simulink model "sim_tank_2_PI"  (R2016b)
settings: Solver=VariableStepAuto  StartTime=0.0  StopTime=10.0  RelTol=1e-3
values from neighbouring files (symbols this model uses):
  Ao1 = pi * Do1^2 / 4    (= 0.17813934812)    [setup_tanks_parameters.m]
  Ao2 = pi * Do2^2 / 4    (= 0.17813934812)    [setup_tanks_parameters.m]
  At1 = pi * Dt1^2 / 4    (= 15.5179165474)    [setup_tanks_parameters.m]
  At2 = pi * Dt2^2 / 4    (= 15.5179165474)    [setup_tanks_parameters.m]
  g = 981    [setup_tanks_parameters.m]
  Ki_1 = Ki1_pp    [d_tanks_1.m]    (also in setup_lab_tanks.m = 0)
  Ki_2 = Ki2_pp    [d_tanks_2.m]    (also in d_tanks_3.m = K(3); setup_lab_tanks.m = 0)
  Kp = 3.3    [setup_tanks_parameters.m]
  Kp_1 = Kp1_pp    [d_tanks_1.m]    (also in d_tanks_3.m = K(1); setup_lab_tanks.m = 0)
  Kp_2 = Kp2_pp    [d_tanks_2.m]    (also in d_tanks_3.m = K(2); setup_lab_tanks.m = 0)
  L20 = L0    [d_tanks_2.m]    (also in setup_lab_tanks.m = 10)
  LR_1_MAX = 25    [setup_lab_tanks.m]
  MAX_L1_WDUP = 3    [setup_lab_tanks.m]
  MAX_L2_WDUP = 3    [setup_lab_tanks.m]
  TS = 35    [setup_lab_tanks.m]
  VMAX_AMP = 22    [setup_tanks_parameters.m]
settings Model: Creator=yuthon  LastModifiedBy=yuthon

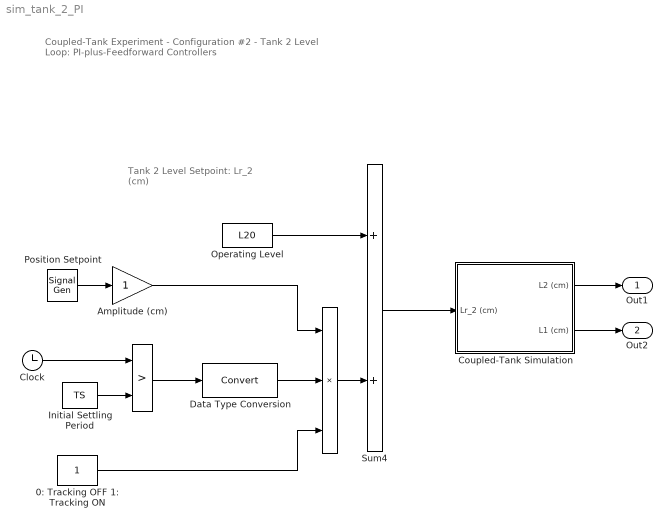
== system sim_tank_2_PI ==
  note: Coupled-Tank Experiment
      | - Configuration #2 -
      | Tank 2 Level Loop:
      | PI-plus-Feedforward Controllers
  note: Tank 2 Level Setpoint:
      | Lr_2 (cm)
  "   " : Product  Inputs=3  SaturateOnIntegerOverflow=on  RndMeth=Zero  InputSameDT=on  OutDataTypeStr=Inherit: Same as first input
  "    " : RelationalOperator  Operator=>  RndMeth=Nearest  InputSameDT=on
  0: Tracking OFF 1: Tracking ON : Constant
  Amplitude (cm) : Gain  SaturateOnIntegerOverflow=on  OutDataTypeStr=Inherit: Same as input  ParamDataTypeStr=Inherit: Same as input
  Clock : Clock
  Coupled-Tank Simulation : Subsystem
  Data Type Conversion : DataTypeConversion
  Initial Settling Period : Constant  Value=TS
  Operating Level : Constant  Value=L20
  Position Setpoint : SignalGenerator  WaveForm=square  Frequency=0.018
  Sum4 : Sum  SaturateOnIntegerOverflow=on  InputSameDT=on  OutDataTypeStr=Inherit: Same as first input
  Out1 : Outport  SignalName=L2  InitialOutput=0
  Out2 : Outport  Port=2  SignalName=L1  InitialOutput=0
  wires:
  Position Setpoint/1 -> Amplitude (cm)/1
  0: Tracking OFF 1: Tracking ON/1 -> "   "/3
  "   "/1 -> Sum4/2
  Operating Level/1 -> Sum4/1
  Initial Settling Period/1 -> "    "/2
  Clock/1 -> "    "/1
  Amplitude (cm)/1 -> "   "/1
  Coupled-Tank Simulation/2(L1 (cm)) -> Out2/1
  "    "/1 -> Data Type Conversion/1
  Data Type Conversion/1 -> "   "/2
  Sum4/1 -> Coupled-Tank Simulation/1(Lr_2 (cm))
  Coupled-Tank Simulation/1(L2 (cm)) -> Out1/1

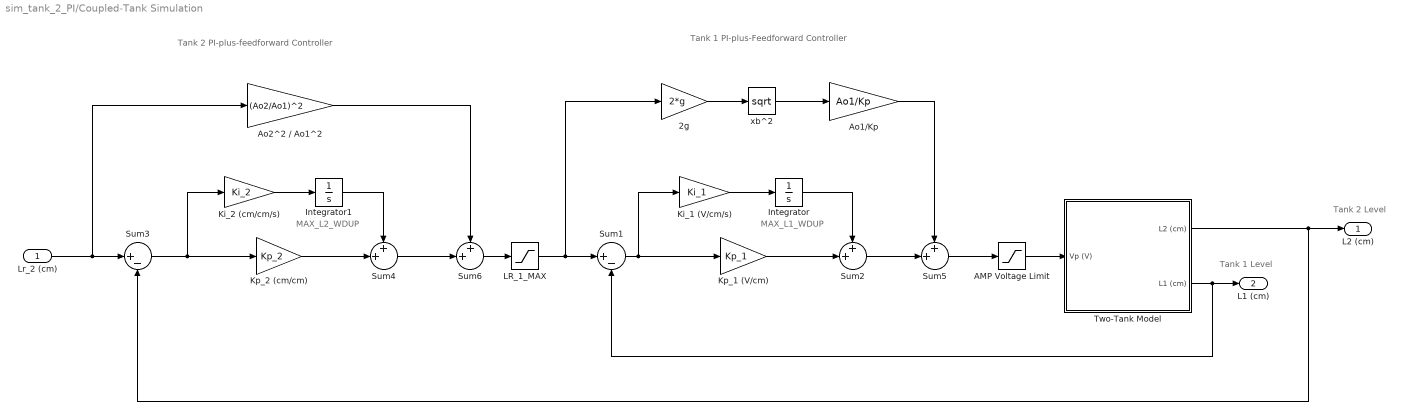
== system sim_tank_2_PI/Coupled-Tank Simulation ==
  note: Tank 1
      | PI-plus-Feedforward Controller
  note: Tank 2
      | PI-plus-feedforward Controller
  note: MAX_L2_WDUP
  note: Tank 1 Level
  note: Tank 2 Level
  note: MAX_L1_WDUP
  Lr_2 (cm) : Inport
  2g : Gain  Gain=2*g  SaturateOnIntegerOverflow=on  OutDataTypeStr=Inherit: Same as input  ParamDataTypeStr=Inherit: Same as input
  AMP Voltage Limit : Saturate  UpperLimit=VMAX_AMP  LowerLimit=0
  Ao1/Kp : Gain  Gain=Ao1/Kp  SaturateOnIntegerOverflow=on  OutDataTypeStr=Inherit: Same as input  ParamDataTypeStr=Inherit: Same as input
  Ao2^2 / Ao1^2 : Gain  Gain=(Ao2/Ao1)^2  SaturateOnIntegerOverflow=on  OutDataTypeStr=Inherit: Same as input  ParamDataTypeStr=Inherit: Same as input
  Integrator : Integrator  LimitOutput=on  UpperSaturationLimit=MAX_L1_WDUP  LowerSaturationLimit=- MAX_L1_WDUP
  Integrator1 : Integrator  LimitOutput=on  UpperSaturationLimit=MAX_L2_WDUP  LowerSaturationLimit=- MAX_L2_WDUP
  Ki_1 (V/cm/s) : Gain  Gain=Ki_1  SaturateOnIntegerOverflow=on  OutDataTypeStr=Inherit: Same as input  ParamDataTypeStr=Inherit: Same as input
  Ki_2 (cm/cm/s) : Gain  Gain=Ki_2  SaturateOnIntegerOverflow=on  OutDataTypeStr=Inherit: Same as input  ParamDataTypeStr=Inherit: Same as input
  Kp_1 (V/cm) : Gain  Gain=Kp_1  SaturateOnIntegerOverflow=on  OutDataTypeStr=Inherit: Same as input  ParamDataTypeStr=Inherit: Same as input
  Kp_2 (cm/cm) : Gain  Gain=Kp_2  SaturateOnIntegerOverflow=on  OutDataTypeStr=Inherit: Same as input  ParamDataTypeStr=Inherit: Same as input
  LR_1_MAX : Saturate  UpperLimit=LR_1_MAX  LowerLimit=0
  Sum1 : Sum  Inputs=|+-  SaturateOnIntegerOverflow=on  InputSameDT=on  OutDataTypeStr=Inherit: Same as first input
  Sum{2,4..6} (4 alike) : Sum  Inputs=++|  SaturateOnIntegerOverflow=on  InputSameDT=on  OutDataTypeStr=Inherit: Same as first input
  Sum3 : Sum  Inputs=|+-  SaturateOnIntegerOverflow=on  InputSameDT=on  OutDataTypeStr=Inherit: Same as first input
  Two-Tank Model : Subsystem
  xb^2 : Math  Operator=sqrt  SaturateOnIntegerOverflow=on
  L2 (cm) : Outport  InitialOutput=0
  L1 (cm) : Outport  Port=2  InitialOutput=0
  wires:
  LR_1_MAX/1 -> 2g/1, Sum1/1
  Lr_2 (cm)/1 -> Ao2^2 / Ao1^2/1, Sum3/1
  Ao2^2 / Ao1^2/1 -> Sum6/1
  Sum6/1 -> LR_1_MAX/1
  Sum4/1 -> Sum6/2
  Integrator1/1 -> Sum4/1
  Kp_2 (cm/cm)/1 -> Sum4/2
  Ki_2 (cm/cm/s)/1 -> Integrator1/1
  Sum3/1 -> Kp_2 (cm/cm)/1, Ki_2 (cm/cm/s)/1
  Two-Tank Model/1(L2 (cm)) -> Sum3/2, L2 (cm)/1
  Two-Tank Model/2(L1 (cm)) -> L1 (cm)/1, Sum1/2
  Ao1/Kp/1 -> Sum5/1
  xb^2/1 -> Ao1/Kp/1
  2g/1 -> xb^2/1
  Sum5/1 -> AMP Voltage Limit/1
  Sum2/1 -> Sum5/2
  AMP Voltage Limit/1 -> Two-Tank Model/1(Vp (V))
  Integrator/1 -> Sum2/1
  Kp_1 (V/cm)/1 -> Sum2/2
  Ki_1 (V/cm/s)/1 -> Integrator/1
  Sum1/1 -> Kp_1 (V/cm)/1, Ki_1 (V/cm/s)/1

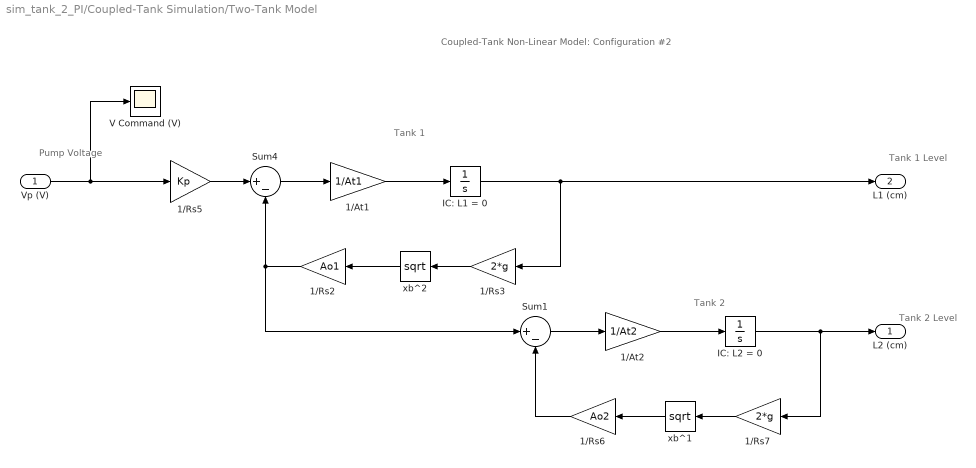
== system sim_tank_2_PI/Coupled-Tank Simulation/Two-Tank Model ==
  note: Pump
      | Voltage
  note: Tank 1 Level
  note: Tank 2 Level
  note: Tank 2
  note: Tank 1
  note: Coupled-Tank Non-Linear Model:
      | Configuration #2
  Vp (V) : Inport
  1/At1 : Gain  Gain=1/At1  SaturateOnIntegerOverflow=on  OutDataTypeStr=Inherit: Same as input  ParamDataTypeStr=Inherit: Same as input
  1/At2 : Gain  Gain=1/At2  SaturateOnIntegerOverflow=on  OutDataTypeStr=Inherit: Same as input  ParamDataTypeStr=Inherit: Same as input
  1/Rs2 : Gain  Gain=Ao1  SaturateOnIntegerOverflow=on  OutDataTypeStr=Inherit: Same as input  ParamDataTypeStr=Inherit: Same as input
  1/Rs3 : Gain  Gain=2*g  SaturateOnIntegerOverflow=on  OutDataTypeStr=Inherit: Same as input  ParamDataTypeStr=Inherit: Same as input
  1/Rs5 : Gain  Gain=Kp  SaturateOnIntegerOverflow=on  OutDataTypeStr=Inherit: Same as input  ParamDataTypeStr=Inherit: Same as input
  1/Rs6 : Gain  Gain=Ao2  SaturateOnIntegerOverflow=on  OutDataTypeStr=Inherit: Same as input  ParamDataTypeStr=Inherit: Same as input
  1/Rs7 : Gain  Gain=2*g  SaturateOnIntegerOverflow=on  OutDataTypeStr=Inherit: Same as input  ParamDataTypeStr=Inherit: Same as input
  IC: L1 = 0 : Integrator
  IC: L2 = 0 : Integrator
  Sum1 : Sum  Inputs=|+-  SaturateOnIntegerOverflow=on  InputSameDT=on  OutDataTypeStr=Inherit: Same as first input
  Sum4 : Sum  Inputs=|+-  SaturateOnIntegerOverflow=on  InputSameDT=on  OutDataTypeStr=Inherit: Same as first input
  V Command (V) : Scope
  xb^1 : Math  Operator=sqrt  SaturateOnIntegerOverflow=on
  xb^2 : Math  Operator=sqrt  SaturateOnIntegerOverflow=on
  L2 (cm) : Outport  InitialOutput=0
  L1 (cm) : Outport  Port=2  InitialOutput=0
  wires:
  1/Rs7/1 -> xb^1/1
  xb^1/1 -> 1/Rs6/1
  1/Rs6/1 -> Sum1/2
  IC: L2 = 0/1 -> L2 (cm)/1, 1/Rs7/1
  1/At2/1 -> IC: L2 = 0/1
  Sum1/1 -> 1/At2/1
  1/Rs3/1 -> xb^2/1
  xb^2/1 -> 1/Rs2/1
  1/Rs2/1 -> Sum1/1, Sum4/2
  IC: L1 = 0/1 -> L1 (cm)/1, 1/Rs3/1
  1/At1/1 -> IC: L1 = 0/1
  Sum4/1 -> 1/At1/1
  1/Rs5/1 -> Sum4/1
  Vp (V)/1 -> 1/Rs5/1, V Command (V)/1
